simulink model "ROCAUC_2016b"  (R2016b)
settings: Solver=VariableStepAuto  StartTime=0.0  StopTime=10.0  RelTol=1e-3
settings Model: Creator=aoki-soya  LastModifiedBy=aoki-soya

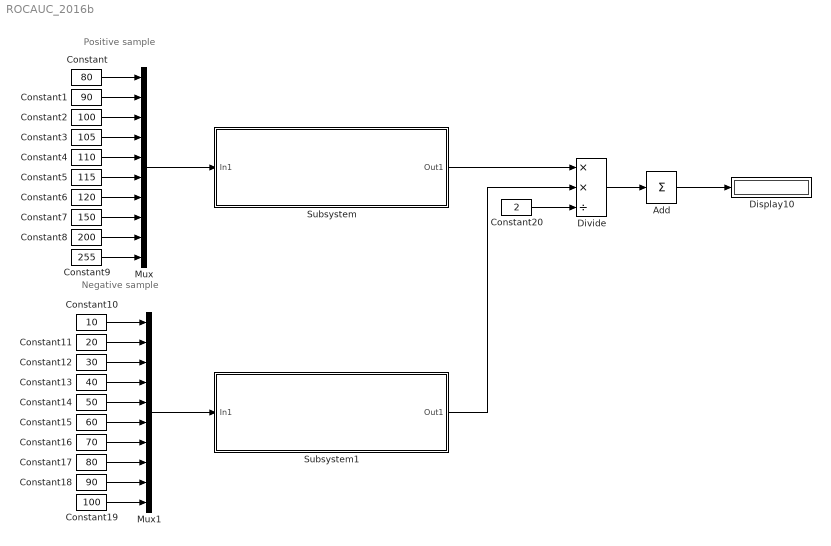
== system ROCAUC_2016b ==
  note: Positive sample
  note: Negative sample
  Add : Sum  Inputs=+
  Constant : Constant  Value=80
  Constant1 : Constant  Value=90
  Constant10 : Constant  Value=10
  Constant11 : Constant  Value=20
  Constant12 : Constant  Value=30
  Constant13 : Constant  Value=40
  Constant14 : Constant  Value=50
  Constant15 : Constant  Value=60
  Constant16 : Constant  Value=70
  Constant17 : Constant  Value=80
  Constant18 : Constant  Value=90
  Constant19 : Constant  Value=100
  Constant2 : Constant  Value=100
  Constant20 : Constant  Value=2
  Constant3 : Constant  Value=105
  Constant4 : Constant  Value=110
  Constant5 : Constant  Value=115
  Constant6 : Constant  Value=120
  Constant7 : Constant  Value=150
  Constant8 : Constant  Value=200
  Constant9 : Constant  Value=255
  Display10 : Display
  Divide : Product  Inputs=**/
  Mux : Mux  Inputs=10
  Mux1 : Mux  Inputs=10
  Subsystem : Subsystem
  Subsystem1 : Subsystem
  wires:
  Constant/1 -> Mux/1
  Constant2/1 -> Mux/3
  Constant1/1 -> Mux/2
  Constant3/1 -> Mux/4
  Constant4/1 -> Mux/5
  Constant5/1 -> Mux/6
  Constant6/1 -> Mux/7
  Constant7/1 -> Mux/8
  Constant8/1 -> Mux/9
  Constant9/1 -> Mux/10
  Constant10/1 -> Mux1/1
  Constant14/1 -> Mux1/5
  Constant13/1 -> Mux1/4
  Constant18/1 -> Mux1/9
  Constant15/1 -> Mux1/6
  Constant16/1 -> Mux1/7
  Constant17/1 -> Mux1/8
  Constant19/1 -> Mux1/10
  Constant11/1 -> Mux1/2
  Constant12/1 -> Mux1/3
  Constant20/1 -> Divide/3
  Mux/1 -> Subsystem/1(In1)
  Mux1/1 -> Subsystem1/1(In1)
  Subsystem/1(Out1) -> Divide/1
  Subsystem1/1(Out1) -> Divide/2
  Divide/1 -> Add/1
  Add/1 -> Display10/1

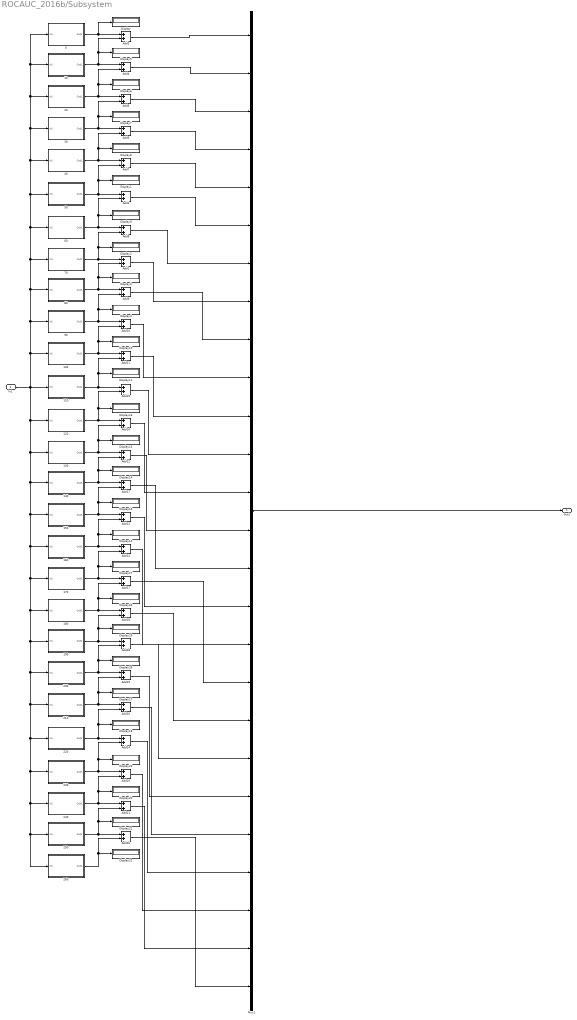
== system ROCAUC_2016b/Subsystem ==
  In1 : Inport
  0 : Subsystem
  10 : Subsystem
  100 : Subsystem
  110 : Subsystem
  120 : Subsystem
  130 : Subsystem
  140 : Subsystem
  150 : Subsystem
  160 : Subsystem
  170 : Subsystem
  180 : Subsystem
  190 : Subsystem
  20 : Subsystem
  200 : Subsystem
  210 : Subsystem
  220 : Subsystem
  230 : Subsystem
  240 : Subsystem
  250 : Subsystem
  260 : Subsystem
  30 : Subsystem
  40 : Subsystem
  50 : Subsystem
  60 : Subsystem
  70 : Subsystem
  80 : Subsystem
  90 : Subsystem
  Add{1..21,24..28} (26 alike) : Sum
  Display{,1..18,20..27} (27 alike) : Display
  Mux2 : Mux  Inputs=26
  Out1 : Outport
  wires:
  0/1(Out1) -> Add3/1, Display/1
  Mux2/1 -> Out1/1
  Add3/1 -> Mux2/1
  50/1(Out1) -> Add7/2, Display1/1, Add2/1
  10/1(Out1) -> Add4/1, Display5/1, Add3/2
  Add4/1 -> Mux2/2
  20/1(Out1) -> Add5/1, Add4/2, Display6/1
  Add5/1 -> Mux2/3
  30/1(Out1) -> Add6/1, Add5/2, Display7/1
  Add6/1 -> Mux2/4
  40/1(Out1) -> Add7/1, Add6/2, Display8/1
  Add7/1 -> Mux2/5
  Add2/1 -> Mux2/6
  60/1(Out1) -> Add8/1, Add2/2, Display9/1
  Add8/1 -> Mux2/7
  90/1(Out1) -> Add10/1, Add9/2, Display4/1
  70/1(Out1) -> Add1/1, Display2/1, Add8/2
  80/1(Out1) -> Add9/1, Display3/1, Add1/2
  100/1(Out1) -> Add11/1, Add10/2, Display10/1
  Add1/1 -> Mux2/8
  Add9/1 -> Mux2/9
  Add10/1 -> Mux2/10
  Add11/1 -> Mux2/11
  130/1(Out1) -> Add12/1, Display13/1, Add16/2
  140/1(Out1) -> Add17/1, Display14/1, Add12/2
  110/1(Out1) -> Add11/2, Display11/1, Add15/1
  160/1(Out1) -> Add14/1, Add13/2, Display12/1
  150/1(Out1) -> Add13/1, Add17/2, Display15/1
  120/1(Out1) -> Add16/1, Add15/2, Display16/1
  Add15/1 -> Mux2/12
  Add16/1 -> Mux2/13
  Add12/1 -> Mux2/14
  Add17/1 -> Mux2/15
  Add13/1 -> Mux2/16
  Add14/1 -> Mux2/17
  210/1(Out1) -> Add20/1, Add19/2, Display17/1
  180/1(Out1) -> Add18/1, Display24/1, Add27/2
  In1/1 -> 260/1(In1), 250/1(In1), 240/1(In1), 230/1(In1), 220/1(In1), 210/1(In1), 200/1(In1), 190/1(In1), 180/1(In1), 170/1(In1), 160/1(In1), 150/1(In1), 140/1(In1), 130/1(In1), 120/1(In1), 100/1(In1), 90/1(In1), 80/1(In1), 70/1(In1), 60/1(In1), 40/1(In1), 30/1(In1), 20/1(In1), 10/1(In1), 0/1(In1), 50/1(In1), 110/1(In1)
  190/1(Out1) -> Add28/1, Display25/1, Add18/2
  240/1(Out1) -> Add21/1, Display20/1, Add25/2
  200/1(Out1) -> Add19/1, Add28/2, Display26/1
  260/1(Out1) -> Add26/2, Display22/1
  220/1(Out1) -> Add20/2, Display18/1, Add24/1
  230/1(Out1) -> Add25/1, Add24/2, Display23/1
  250/1(Out1) -> Add26/1, Display21/1, Add21/2
  170/1(Out1) -> Add27/1, Add14/2, Display27/1
  Add27/1 -> Mux2/18
  Add18/1 -> Mux2/19
  Add28/1 -> Mux2/20
  Add19/1 -> Mux2/21
  Add26/1 -> Mux2/26
  Add21/1 -> Mux2/25
  Add25/1 -> Mux2/24
  Add24/1 -> Mux2/23
  Add20/1 -> Mux2/22

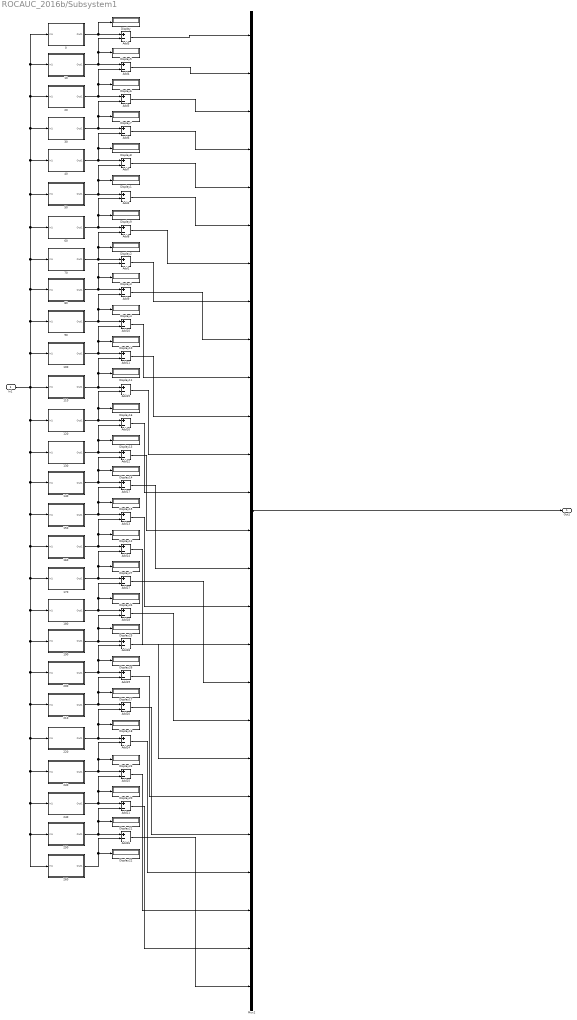
== system ROCAUC_2016b/Subsystem1 ==
  In1 : Inport
  0 : Subsystem
  10 : Subsystem
  100 : Subsystem
  110 : Subsystem
  120 : Subsystem
  130 : Subsystem
  140 : Subsystem
  150 : Subsystem
  160 : Subsystem
  170 : Subsystem
  180 : Subsystem
  190 : Subsystem
  20 : Subsystem
  200 : Subsystem
  210 : Subsystem
  220 : Subsystem
  230 : Subsystem
  240 : Subsystem
  250 : Subsystem
  260 : Subsystem
  30 : Subsystem
  40 : Subsystem
  50 : Subsystem
  60 : Subsystem
  70 : Subsystem
  80 : Subsystem
  90 : Subsystem
  Add{1..21,24..28} (26 alike) : Sum  Inputs=+-
  Display{,1..18,20..27} (27 alike) : Display
  Mux2 : Mux  Inputs=26
  Out1 : Outport
  wires:
  0/1(Out1) -> Add3/1, Display/1
  Mux2/1 -> Out1/1
  Add3/1 -> Mux2/1
  50/1(Out1) -> Add7/2, Display1/1, Add2/1
  10/1(Out1) -> Add4/1, Display5/1, Add3/2
  Add4/1 -> Mux2/2
  20/1(Out1) -> Add5/1, Add4/2, Display6/1
  Add5/1 -> Mux2/3
  30/1(Out1) -> Add6/1, Add5/2, Display7/1
  Add6/1 -> Mux2/4
  40/1(Out1) -> Add7/1, Add6/2, Display8/1
  Add7/1 -> Mux2/5
  Add2/1 -> Mux2/6
  60/1(Out1) -> Add8/1, Add2/2, Display9/1
  Add8/1 -> Mux2/7
  90/1(Out1) -> Add10/1, Add9/2, Display4/1
  70/1(Out1) -> Add1/1, Display2/1, Add8/2
  80/1(Out1) -> Add9/1, Display3/1, Add1/2
  100/1(Out1) -> Add11/1, Add10/2, Display10/1
  Add1/1 -> Mux2/8
  Add9/1 -> Mux2/9
  Add10/1 -> Mux2/10
  Add11/1 -> Mux2/11
  130/1(Out1) -> Add12/1, Display13/1, Add16/2
  140/1(Out1) -> Add17/1, Display14/1, Add12/2
  110/1(Out1) -> Add11/2, Display11/1, Add15/1
  160/1(Out1) -> Add14/1, Add13/2, Display12/1
  150/1(Out1) -> Add13/1, Add17/2, Display15/1
  120/1(Out1) -> Add16/1, Add15/2, Display16/1
  Add15/1 -> Mux2/12
  Add16/1 -> Mux2/13
  Add12/1 -> Mux2/14
  Add17/1 -> Mux2/15
  Add13/1 -> Mux2/16
  Add14/1 -> Mux2/17
  210/1(Out1) -> Add20/1, Add19/2, Display17/1
  180/1(Out1) -> Add18/1, Display24/1, Add27/2
  In1/1 -> 260/1(In1), 250/1(In1), 240/1(In1), 230/1(In1), 220/1(In1), 210/1(In1), 200/1(In1), 190/1(In1), 180/1(In1), 170/1(In1), 160/1(In1), 150/1(In1), 140/1(In1), 130/1(In1), 120/1(In1), 100/1(In1), 90/1(In1), 80/1(In1), 70/1(In1), 60/1(In1), 40/1(In1), 30/1(In1), 20/1(In1), 10/1(In1), 0/1(In1), 50/1(In1), 110/1(In1)
  190/1(Out1) -> Add28/1, Display25/1, Add18/2
  240/1(Out1) -> Add21/1, Display20/1, Add25/2
  200/1(Out1) -> Add19/1, Add28/2, Display26/1
  260/1(Out1) -> Add26/2, Display22/1
  220/1(Out1) -> Add20/2, Display18/1, Add24/1
  230/1(Out1) -> Add25/1, Add24/2, Display23/1
  250/1(Out1) -> Add26/1, Display21/1, Add21/2
  170/1(Out1) -> Add27/1, Add14/2, Display27/1
  Add27/1 -> Mux2/18
  Add18/1 -> Mux2/19
  Add28/1 -> Mux2/20
  Add19/1 -> Mux2/21
  Add26/1 -> Mux2/26
  Add21/1 -> Mux2/25
  Add25/1 -> Mux2/24
  Add24/1 -> Mux2/23
  Add20/1 -> Mux2/22

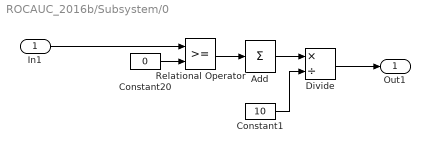
== system ROCAUC_2016b/Subsystem/0 ==
  In1 : Inport
  Add : Sum  Inputs=+
  Constant1 : Constant  Value=10
  Constant20 : Constant  Value=0
  Divide : Product  Inputs=*/
  Relational Operator : RelationalOperator  OutDataTypeStr=boolean  RndMeth=Simplest
  Out1 : Outport
  wires:
  Constant20/1 -> Relational Operator/2
  Relational Operator/1 -> Add/1
  In1/1 -> Relational Operator/1
  Add/1 -> Divide/1
  Divide/1 -> Out1/1
  Constant1/1 -> Divide/2

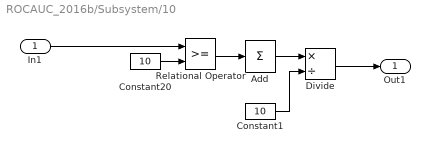
== system ROCAUC_2016b/Subsystem/10 ==
  In1 : Inport
  Add : Sum  Inputs=+
  Constant1 : Constant  Value=10
  Constant20 : Constant  Value=10
  Divide : Product  Inputs=*/
  Relational Operator : RelationalOperator  OutDataTypeStr=boolean  RndMeth=Simplest
  Out1 : Outport
  wires:
  Constant20/1 -> Relational Operator/2
  Relational Operator/1 -> Add/1
  In1/1 -> Relational Operator/1
  Add/1 -> Divide/1
  Divide/1 -> Out1/1
  Constant1/1 -> Divide/2

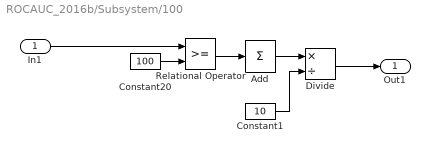
== system ROCAUC_2016b/Subsystem/100 ==
  In1 : Inport
  Add : Sum  Inputs=+
  Constant1 : Constant  Value=10
  Constant20 : Constant  Value=100
  Divide : Product  Inputs=*/
  Relational Operator : RelationalOperator  OutDataTypeStr=boolean  RndMeth=Simplest
  Out1 : Outport
  wires:
  Constant20/1 -> Relational Operator/2
  Relational Operator/1 -> Add/1
  In1/1 -> Relational Operator/1
  Add/1 -> Divide/1
  Divide/1 -> Out1/1
  Constant1/1 -> Divide/2

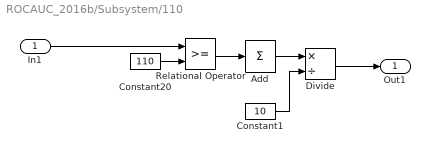
== system ROCAUC_2016b/Subsystem/110 ==
  In1 : Inport
  Add : Sum  Inputs=+
  Constant1 : Constant  Value=10
  Constant20 : Constant  Value=110
  Divide : Product  Inputs=*/
  Relational Operator : RelationalOperator  OutDataTypeStr=boolean  RndMeth=Simplest
  Out1 : Outport
  wires:
  In1/1 -> Relational Operator/1
  Relational Operator/1 -> Add/1
  Constant1/1 -> Divide/2
  Add/1 -> Divide/1
  Constant20/1 -> Relational Operator/2
  Divide/1 -> Out1/1

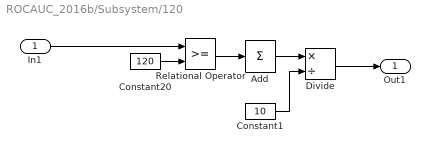
== system ROCAUC_2016b/Subsystem/120 ==
  In1 : Inport
  Add : Sum  Inputs=+
  Constant1 : Constant  Value=10
  Constant20 : Constant  Value=120
  Divide : Product  Inputs=*/
  Relational Operator : RelationalOperator  OutDataTypeStr=boolean  RndMeth=Simplest
  Out1 : Outport
  wires:
  Constant20/1 -> Relational Operator/2
  Relational Operator/1 -> Add/1
  In1/1 -> Relational Operator/1
  Add/1 -> Divide/1
  Divide/1 -> Out1/1
  Constant1/1 -> Divide/2

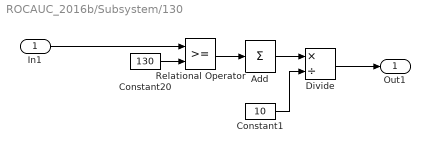
== system ROCAUC_2016b/Subsystem/130 ==
  In1 : Inport
  Add : Sum  Inputs=+
  Constant1 : Constant  Value=10
  Constant20 : Constant  Value=130
  Divide : Product  Inputs=*/
  Relational Operator : RelationalOperator  OutDataTypeStr=boolean  RndMeth=Simplest
  Out1 : Outport
  wires:
  Constant20/1 -> Relational Operator/2
  Relational Operator/1 -> Add/1
  In1/1 -> Relational Operator/1
  Add/1 -> Divide/1
  Divide/1 -> Out1/1
  Constant1/1 -> Divide/2

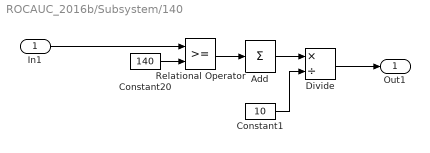
== system ROCAUC_2016b/Subsystem/140 ==
  In1 : Inport
  Add : Sum  Inputs=+
  Constant1 : Constant  Value=10
  Constant20 : Constant  Value=140
  Divide : Product  Inputs=*/
  Relational Operator : RelationalOperator  OutDataTypeStr=boolean  RndMeth=Simplest
  Out1 : Outport
  wires:
  Constant20/1 -> Relational Operator/2
  Relational Operator/1 -> Add/1
  In1/1 -> Relational Operator/1
  Add/1 -> Divide/1
  Divide/1 -> Out1/1
  Constant1/1 -> Divide/2

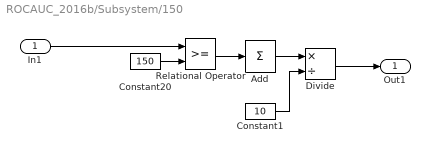
== system ROCAUC_2016b/Subsystem/150 ==
  In1 : Inport
  Add : Sum  Inputs=+
  Constant1 : Constant  Value=10
  Constant20 : Constant  Value=150
  Divide : Product  Inputs=*/
  Relational Operator : RelationalOperator  OutDataTypeStr=boolean  RndMeth=Simplest
  Out1 : Outport
  wires:
  Constant20/1 -> Relational Operator/2
  Relational Operator/1 -> Add/1
  In1/1 -> Relational Operator/1
  Add/1 -> Divide/1
  Divide/1 -> Out1/1
  Constant1/1 -> Divide/2

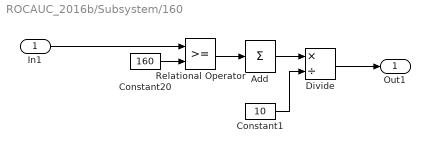
== system ROCAUC_2016b/Subsystem/160 ==
  In1 : Inport
  Add : Sum  Inputs=+
  Constant1 : Constant  Value=10
  Constant20 : Constant  Value=160
  Divide : Product  Inputs=*/
  Relational Operator : RelationalOperator  OutDataTypeStr=boolean  RndMeth=Simplest
  Out1 : Outport
  wires:
  Constant20/1 -> Relational Operator/2
  Relational Operator/1 -> Add/1
  In1/1 -> Relational Operator/1
  Add/1 -> Divide/1
  Divide/1 -> Out1/1
  Constant1/1 -> Divide/2

== system ROCAUC_2016b/Subsystem/170 ==
  In1 : Inport
  Add : Sum  Inputs=+
  Constant1 : Constant  Value=10
  Constant20 : Constant  Value=170
  Divide : Product  Inputs=*/
  Relational Operator : RelationalOperator  OutDataTypeStr=boolean  RndMeth=Simplest
  Out1 : Outport
  wires:
  Constant20/1 -> Relational Operator/2
  Relational Operator/1 -> Add/1
  In1/1 -> Relational Operator/1
  Add/1 -> Divide/1
  Divide/1 -> Out1/1
  Constant1/1 -> Divide/2

== system ROCAUC_2016b/Subsystem/180 ==
  In1 : Inport
  Add : Sum  Inputs=+
  Constant1 : Constant  Value=10
  Constant20 : Constant  Value=180
  Divide : Product  Inputs=*/
  Relational Operator : RelationalOperator  OutDataTypeStr=boolean  RndMeth=Simplest
  Out1 : Outport
  wires:
  Constant20/1 -> Relational Operator/2
  Relational Operator/1 -> Add/1
  In1/1 -> Relational Operator/1
  Add/1 -> Divide/1
  Divide/1 -> Out1/1
  Constant1/1 -> Divide/2

== system ROCAUC_2016b/Subsystem/190 ==
  In1 : Inport
  Add : Sum  Inputs=+
  Constant1 : Constant  Value=10
  Constant20 : Constant  Value=190
  Divide : Product  Inputs=*/
  Relational Operator : RelationalOperator  OutDataTypeStr=boolean  RndMeth=Simplest
  Out1 : Outport
  wires:
  Constant20/1 -> Relational Operator/2
  Relational Operator/1 -> Add/1
  In1/1 -> Relational Operator/1
  Add/1 -> Divide/1
  Divide/1 -> Out1/1
  Constant1/1 -> Divide/2

== system ROCAUC_2016b/Subsystem/20 ==
  In1 : Inport
  Add : Sum  Inputs=+
  Constant1 : Constant  Value=10
  Constant20 : Constant  Value=20
  Divide : Product  Inputs=*/
  Relational Operator : RelationalOperator  OutDataTypeStr=boolean  RndMeth=Simplest
  Out1 : Outport
  wires:
  Constant20/1 -> Relational Operator/2
  Relational Operator/1 -> Add/1
  In1/1 -> Relational Operator/1
  Add/1 -> Divide/1
  Divide/1 -> Out1/1
  Constant1/1 -> Divide/2

== system ROCAUC_2016b/Subsystem/200 ==
  In1 : Inport
  Add : Sum  Inputs=+
  Constant1 : Constant  Value=10
  Constant20 : Constant  Value=200
  Divide : Product  Inputs=*/
  Relational Operator : RelationalOperator  OutDataTypeStr=boolean  RndMeth=Simplest
  Out1 : Outport
  wires:
  Constant20/1 -> Relational Operator/2
  Relational Operator/1 -> Add/1
  In1/1 -> Relational Operator/1
  Add/1 -> Divide/1
  Divide/1 -> Out1/1
  Constant1/1 -> Divide/2

== system ROCAUC_2016b/Subsystem/210 ==
  In1 : Inport
  Add : Sum  Inputs=+
  Constant1 : Constant  Value=10
  Constant20 : Constant  Value=210
  Divide : Product  Inputs=*/
  Relational Operator : RelationalOperator  OutDataTypeStr=boolean  RndMeth=Simplest
  Out1 : Outport
  wires:
  Constant20/1 -> Relational Operator/2
  Relational Operator/1 -> Add/1
  In1/1 -> Relational Operator/1
  Add/1 -> Divide/1
  Divide/1 -> Out1/1
  Constant1/1 -> Divide/2

== system ROCAUC_2016b/Subsystem/220 ==
  In1 : Inport
  Add : Sum  Inputs=+
  Constant1 : Constant  Value=10
  Constant20 : Constant  Value=220
  Divide : Product  Inputs=*/
  Relational Operator : RelationalOperator  OutDataTypeStr=boolean  RndMeth=Simplest
  Out1 : Outport
  wires:
  In1/1 -> Relational Operator/1
  Relational Operator/1 -> Add/1
  Constant1/1 -> Divide/2
  Add/1 -> Divide/1
  Constant20/1 -> Relational Operator/2
  Divide/1 -> Out1/1

== system ROCAUC_2016b/Subsystem/230 ==
  In1 : Inport
  Add : Sum  Inputs=+
  Constant1 : Constant  Value=10
  Constant20 : Constant  Value=230
  Divide : Product  Inputs=*/
  Relational Operator : RelationalOperator  OutDataTypeStr=boolean  RndMeth=Simplest
  Out1 : Outport
  wires:
  Constant20/1 -> Relational Operator/2
  Relational Operator/1 -> Add/1
  In1/1 -> Relational Operator/1
  Add/1 -> Divide/1
  Divide/1 -> Out1/1
  Constant1/1 -> Divide/2

== system ROCAUC_2016b/Subsystem/240 ==
  In1 : Inport
  Add : Sum  Inputs=+
  Constant1 : Constant  Value=10
  Constant20 : Constant  Value=240
  Divide : Product  Inputs=*/
  Relational Operator : RelationalOperator  OutDataTypeStr=boolean  RndMeth=Simplest
  Out1 : Outport
  wires:
  Constant20/1 -> Relational Operator/2
  Relational Operator/1 -> Add/1
  In1/1 -> Relational Operator/1
  Add/1 -> Divide/1
  Divide/1 -> Out1/1
  Constant1/1 -> Divide/2

== system ROCAUC_2016b/Subsystem/250 ==
  In1 : Inport
  Add : Sum  Inputs=+
  Constant1 : Constant  Value=10
  Constant20 : Constant  Value=250
  Divide : Product  Inputs=*/
  Relational Operator : RelationalOperator  OutDataTypeStr=boolean  RndMeth=Simplest
  Out1 : Outport
  wires:
  Constant20/1 -> Relational Operator/2
  Relational Operator/1 -> Add/1
  In1/1 -> Relational Operator/1
  Add/1 -> Divide/1
  Divide/1 -> Out1/1
  Constant1/1 -> Divide/2

== system ROCAUC_2016b/Subsystem/260 ==
  In1 : Inport
  Add : Sum  Inputs=+
  Constant1 : Constant  Value=10
  Constant20 : Constant  Value=260
  Divide : Product  Inputs=*/
  Relational Operator : RelationalOperator  OutDataTypeStr=boolean  RndMeth=Simplest
  Out1 : Outport
  wires:
  Constant20/1 -> Relational Operator/2
  Relational Operator/1 -> Add/1
  In1/1 -> Relational Operator/1
  Add/1 -> Divide/1
  Divide/1 -> Out1/1
  Constant1/1 -> Divide/2

== system ROCAUC_2016b/Subsystem/30 ==
  In1 : Inport
  Add : Sum  Inputs=+
  Constant1 : Constant  Value=10
  Constant20 : Constant  Value=30
  Divide : Product  Inputs=*/
  Relational Operator : RelationalOperator  OutDataTypeStr=boolean  RndMeth=Simplest
  Out1 : Outport
  wires:
  Constant20/1 -> Relational Operator/2
  Relational Operator/1 -> Add/1
  In1/1 -> Relational Operator/1
  Add/1 -> Divide/1
  Divide/1 -> Out1/1
  Constant1/1 -> Divide/2

== system ROCAUC_2016b/Subsystem/40 ==
  In1 : Inport
  Add : Sum  Inputs=+
  Constant1 : Constant  Value=10
  Constant20 : Constant  Value=40
  Divide : Product  Inputs=*/
  Relational Operator : RelationalOperator  OutDataTypeStr=boolean  RndMeth=Simplest
  Out1 : Outport
  wires:
  Constant20/1 -> Relational Operator/2
  Relational Operator/1 -> Add/1
  In1/1 -> Relational Operator/1
  Add/1 -> Divide/1
  Divide/1 -> Out1/1
  Constant1/1 -> Divide/2

== system ROCAUC_2016b/Subsystem/50 ==
  In1 : Inport
  Add : Sum  Inputs=+
  Constant1 : Constant  Value=10
  Constant20 : Constant  Value=50
  Divide : Product  Inputs=*/
  Relational Operator : RelationalOperator  OutDataTypeStr=boolean  RndMeth=Simplest
  Out1 : Outport
  wires:
  In1/1 -> Relational Operator/1
  Relational Operator/1 -> Add/1
  Constant1/1 -> Divide/2
  Add/1 -> Divide/1
  Constant20/1 -> Relational Operator/2
  Divide/1 -> Out1/1

== system ROCAUC_2016b/Subsystem/60 ==
  In1 : Inport
  Add : Sum  Inputs=+
  Constant1 : Constant  Value=10
  Constant20 : Constant  Value=60
  Divide : Product  Inputs=*/
  Relational Operator : RelationalOperator  OutDataTypeStr=boolean  RndMeth=Simplest
  Out1 : Outport
  wires:
  Constant20/1 -> Relational Operator/2
  Relational Operator/1 -> Add/1
  In1/1 -> Relational Operator/1
  Add/1 -> Divide/1
  Divide/1 -> Out1/1
  Constant1/1 -> Divide/2

== system ROCAUC_2016b/Subsystem/70 ==
  In1 : Inport
  Add : Sum  Inputs=+
  Constant1 : Constant  Value=10
  Constant20 : Constant  Value=70
  Divide : Product  Inputs=*/
  Relational Operator : RelationalOperator  OutDataTypeStr=boolean  RndMeth=Simplest
  Out1 : Outport
  wires:
  Constant20/1 -> Relational Operator/2
  Relational Operator/1 -> Add/1
  In1/1 -> Relational Operator/1
  Add/1 -> Divide/1
  Divide/1 -> Out1/1
  Constant1/1 -> Divide/2

== system ROCAUC_2016b/Subsystem/80 ==
  In1 : Inport
  Add : Sum  Inputs=+
  Constant1 : Constant  Value=10
  Constant20 : Constant  Value=80
  Divide : Product  Inputs=*/
  Relational Operator : RelationalOperator  OutDataTypeStr=boolean  RndMeth=Simplest
  Out1 : Outport
  wires:
  Constant20/1 -> Relational Operator/2
  Relational Operator/1 -> Add/1
  In1/1 -> Relational Operator/1
  Add/1 -> Divide/1
  Divide/1 -> Out1/1
  Constant1/1 -> Divide/2

== system ROCAUC_2016b/Subsystem/90 ==
  In1 : Inport
  Add : Sum  Inputs=+
  Constant1 : Constant  Value=10
  Constant20 : Constant  Value=90
  Divide : Product  Inputs=*/
  Relational Operator : RelationalOperator  OutDataTypeStr=boolean  RndMeth=Simplest
  Out1 : Outport
  wires:
  Constant20/1 -> Relational Operator/2
  Relational Operator/1 -> Add/1
  In1/1 -> Relational Operator/1
  Add/1 -> Divide/1
  Divide/1 -> Out1/1
  Constant1/1 -> Divide/2

== system ROCAUC_2016b/Subsystem1/0 ==
  In1 : Inport
  Add : Sum  Inputs=+
  Constant1 : Constant  Value=10
  Constant20 : Constant  Value=0
  Divide : Product  Inputs=*/
  Relational Operator : RelationalOperator  OutDataTypeStr=boolean  RndMeth=Simplest
  Out1 : Outport
  wires:
  Constant20/1 -> Relational Operator/2
  Relational Operator/1 -> Add/1
  In1/1 -> Relational Operator/1
  Add/1 -> Divide/1
  Divide/1 -> Out1/1
  Constant1/1 -> Divide/2

== system ROCAUC_2016b/Subsystem1/10 ==
  In1 : Inport
  Add : Sum  Inputs=+
  Constant1 : Constant  Value=10
  Constant20 : Constant  Value=10
  Divide : Product  Inputs=*/
  Relational Operator : RelationalOperator  OutDataTypeStr=boolean  RndMeth=Simplest
  Out1 : Outport
  wires:
  Constant20/1 -> Relational Operator/2
  Relational Operator/1 -> Add/1
  In1/1 -> Relational Operator/1
  Add/1 -> Divide/1
  Divide/1 -> Out1/1
  Constant1/1 -> Divide/2

== system ROCAUC_2016b/Subsystem1/100 ==
  In1 : Inport
  Add : Sum  Inputs=+
  Constant1 : Constant  Value=10
  Constant20 : Constant  Value=100
  Divide : Product  Inputs=*/
  Relational Operator : RelationalOperator  OutDataTypeStr=boolean  RndMeth=Simplest
  Out1 : Outport
  wires:
  Constant20/1 -> Relational Operator/2
  Relational Operator/1 -> Add/1
  In1/1 -> Relational Operator/1
  Add/1 -> Divide/1
  Divide/1 -> Out1/1
  Constant1/1 -> Divide/2

== system ROCAUC_2016b/Subsystem1/110 ==
  In1 : Inport
  Add : Sum  Inputs=+
  Constant1 : Constant  Value=10
  Constant20 : Constant  Value=110
  Divide : Product  Inputs=*/
  Relational Operator : RelationalOperator  OutDataTypeStr=boolean  RndMeth=Simplest
  Out1 : Outport
  wires:
  In1/1 -> Relational Operator/1
  Relational Operator/1 -> Add/1
  Constant1/1 -> Divide/2
  Add/1 -> Divide/1
  Constant20/1 -> Relational Operator/2
  Divide/1 -> Out1/1

== system ROCAUC_2016b/Subsystem1/120 ==
  In1 : Inport
  Add : Sum  Inputs=+
  Constant1 : Constant  Value=10
  Constant20 : Constant  Value=120
  Divide : Product  Inputs=*/
  Relational Operator : RelationalOperator  OutDataTypeStr=boolean  RndMeth=Simplest
  Out1 : Outport
  wires:
  Constant20/1 -> Relational Operator/2
  Relational Operator/1 -> Add/1
  In1/1 -> Relational Operator/1
  Add/1 -> Divide/1
  Divide/1 -> Out1/1
  Constant1/1 -> Divide/2

== system ROCAUC_2016b/Subsystem1/130 ==
  In1 : Inport
  Add : Sum  Inputs=+
  Constant1 : Constant  Value=10
  Constant20 : Constant  Value=130
  Divide : Product  Inputs=*/
  Relational Operator : RelationalOperator  OutDataTypeStr=boolean  RndMeth=Simplest
  Out1 : Outport
  wires:
  Constant20/1 -> Relational Operator/2
  Relational Operator/1 -> Add/1
  In1/1 -> Relational Operator/1
  Add/1 -> Divide/1
  Divide/1 -> Out1/1
  Constant1/1 -> Divide/2

== system ROCAUC_2016b/Subsystem1/140 ==
  In1 : Inport
  Add : Sum  Inputs=+
  Constant1 : Constant  Value=10
  Constant20 : Constant  Value=140
  Divide : Product  Inputs=*/
  Relational Operator : RelationalOperator  OutDataTypeStr=boolean  RndMeth=Simplest
  Out1 : Outport
  wires:
  Constant20/1 -> Relational Operator/2
  Relational Operator/1 -> Add/1
  In1/1 -> Relational Operator/1
  Add/1 -> Divide/1
  Divide/1 -> Out1/1
  Constant1/1 -> Divide/2

== system ROCAUC_2016b/Subsystem1/150 ==
  In1 : Inport
  Add : Sum  Inputs=+
  Constant1 : Constant  Value=10
  Constant20 : Constant  Value=150
  Divide : Product  Inputs=*/
  Relational Operator : RelationalOperator  OutDataTypeStr=boolean  RndMeth=Simplest
  Out1 : Outport
  wires:
  Constant20/1 -> Relational Operator/2
  Relational Operator/1 -> Add/1
  In1/1 -> Relational Operator/1
  Add/1 -> Divide/1
  Divide/1 -> Out1/1
  Constant1/1 -> Divide/2

== system ROCAUC_2016b/Subsystem1/160 ==
  In1 : Inport
  Add : Sum  Inputs=+
  Constant1 : Constant  Value=10
  Constant20 : Constant  Value=160
  Divide : Product  Inputs=*/
  Relational Operator : RelationalOperator  OutDataTypeStr=boolean  RndMeth=Simplest
  Out1 : Outport
  wires:
  Constant20/1 -> Relational Operator/2
  Relational Operator/1 -> Add/1
  In1/1 -> Relational Operator/1
  Add/1 -> Divide/1
  Divide/1 -> Out1/1
  Constant1/1 -> Divide/2

== system ROCAUC_2016b/Subsystem1/170 ==
  In1 : Inport
  Add : Sum  Inputs=+
  Constant1 : Constant  Value=10
  Constant20 : Constant  Value=170
  Divide : Product  Inputs=*/
  Relational Operator : RelationalOperator  OutDataTypeStr=boolean  RndMeth=Simplest
  Out1 : Outport
  wires:
  Constant20/1 -> Relational Operator/2
  Relational Operator/1 -> Add/1
  In1/1 -> Relational Operator/1
  Add/1 -> Divide/1
  Divide/1 -> Out1/1
  Constant1/1 -> Divide/2

== system ROCAUC_2016b/Subsystem1/180 ==
  In1 : Inport
  Add : Sum  Inputs=+
  Constant1 : Constant  Value=10
  Constant20 : Constant  Value=180
  Divide : Product  Inputs=*/
  Relational Operator : RelationalOperator  OutDataTypeStr=boolean  RndMeth=Simplest
  Out1 : Outport
  wires:
  Constant20/1 -> Relational Operator/2
  Relational Operator/1 -> Add/1
  In1/1 -> Relational Operator/1
  Add/1 -> Divide/1
  Divide/1 -> Out1/1
  Constant1/1 -> Divide/2

== system ROCAUC_2016b/Subsystem1/190 ==
  In1 : Inport
  Add : Sum  Inputs=+
  Constant1 : Constant  Value=10
  Constant20 : Constant  Value=190
  Divide : Product  Inputs=*/
  Relational Operator : RelationalOperator  OutDataTypeStr=boolean  RndMeth=Simplest
  Out1 : Outport
  wires:
  Constant20/1 -> Relational Operator/2
  Relational Operator/1 -> Add/1
  In1/1 -> Relational Operator/1
  Add/1 -> Divide/1
  Divide/1 -> Out1/1
  Constant1/1 -> Divide/2

== system ROCAUC_2016b/Subsystem1/20 ==
  In1 : Inport
  Add : Sum  Inputs=+
  Constant1 : Constant  Value=10
  Constant20 : Constant  Value=20
  Divide : Product  Inputs=*/
  Relational Operator : RelationalOperator  OutDataTypeStr=boolean  RndMeth=Simplest
  Out1 : Outport
  wires:
  Constant20/1 -> Relational Operator/2
  Relational Operator/1 -> Add/1
  In1/1 -> Relational Operator/1
  Add/1 -> Divide/1
  Divide/1 -> Out1/1
  Constant1/1 -> Divide/2

== system ROCAUC_2016b/Subsystem1/200 ==
  In1 : Inport
  Add : Sum  Inputs=+
  Constant1 : Constant  Value=10
  Constant20 : Constant  Value=200
  Divide : Product  Inputs=*/
  Relational Operator : RelationalOperator  OutDataTypeStr=boolean  RndMeth=Simplest
  Out1 : Outport
  wires:
  Constant20/1 -> Relational Operator/2
  Relational Operator/1 -> Add/1
  In1/1 -> Relational Operator/1
  Add/1 -> Divide/1
  Divide/1 -> Out1/1
  Constant1/1 -> Divide/2

== system ROCAUC_2016b/Subsystem1/210 ==
  In1 : Inport
  Add : Sum  Inputs=+
  Constant1 : Constant  Value=10
  Constant20 : Constant  Value=210
  Divide : Product  Inputs=*/
  Relational Operator : RelationalOperator  OutDataTypeStr=boolean  RndMeth=Simplest
  Out1 : Outport
  wires:
  Constant20/1 -> Relational Operator/2
  Relational Operator/1 -> Add/1
  In1/1 -> Relational Operator/1
  Add/1 -> Divide/1
  Divide/1 -> Out1/1
  Constant1/1 -> Divide/2

== system ROCAUC_2016b/Subsystem1/220 ==
  In1 : Inport
  Add : Sum  Inputs=+
  Constant1 : Constant  Value=10
  Constant20 : Constant  Value=220
  Divide : Product  Inputs=*/
  Relational Operator : RelationalOperator  OutDataTypeStr=boolean  RndMeth=Simplest
  Out1 : Outport
  wires:
  In1/1 -> Relational Operator/1
  Relational Operator/1 -> Add/1
  Constant1/1 -> Divide/2
  Add/1 -> Divide/1
  Constant20/1 -> Relational Operator/2
  Divide/1 -> Out1/1

== system ROCAUC_2016b/Subsystem1/230 ==
  In1 : Inport
  Add : Sum  Inputs=+
  Constant1 : Constant  Value=10
  Constant20 : Constant  Value=230
  Divide : Product  Inputs=*/
  Relational Operator : RelationalOperator  OutDataTypeStr=boolean  RndMeth=Simplest
  Out1 : Outport
  wires:
  Constant20/1 -> Relational Operator/2
  Relational Operator/1 -> Add/1
  In1/1 -> Relational Operator/1
  Add/1 -> Divide/1
  Divide/1 -> Out1/1
  Constant1/1 -> Divide/2

== system ROCAUC_2016b/Subsystem1/240 ==
  In1 : Inport
  Add : Sum  Inputs=+
  Constant1 : Constant  Value=10
  Constant20 : Constant  Value=240
  Divide : Product  Inputs=*/
  Relational Operator : RelationalOperator  OutDataTypeStr=boolean  RndMeth=Simplest
  Out1 : Outport
  wires:
  Constant20/1 -> Relational Operator/2
  Relational Operator/1 -> Add/1
  In1/1 -> Relational Operator/1
  Add/1 -> Divide/1
  Divide/1 -> Out1/1
  Constant1/1 -> Divide/2

== system ROCAUC_2016b/Subsystem1/250 ==
  In1 : Inport
  Add : Sum  Inputs=+
  Constant1 : Constant  Value=10
  Constant20 : Constant  Value=250
  Divide : Product  Inputs=*/
  Relational Operator : RelationalOperator  OutDataTypeStr=boolean  RndMeth=Simplest
  Out1 : Outport
  wires:
  Constant20/1 -> Relational Operator/2
  Relational Operator/1 -> Add/1
  In1/1 -> Relational Operator/1
  Add/1 -> Divide/1
  Divide/1 -> Out1/1
  Constant1/1 -> Divide/2

== system ROCAUC_2016b/Subsystem1/260 ==
  In1 : Inport
  Add : Sum  Inputs=+
  Constant1 : Constant  Value=10
  Constant20 : Constant  Value=260
  Divide : Product  Inputs=*/
  Relational Operator : RelationalOperator  OutDataTypeStr=boolean  RndMeth=Simplest
  Out1 : Outport
  wires:
  Constant20/1 -> Relational Operator/2
  Relational Operator/1 -> Add/1
  In1/1 -> Relational Operator/1
  Add/1 -> Divide/1
  Divide/1 -> Out1/1
  Constant1/1 -> Divide/2

== system ROCAUC_2016b/Subsystem1/30 ==
  In1 : Inport
  Add : Sum  Inputs=+
  Constant1 : Constant  Value=10
  Constant20 : Constant  Value=30
  Divide : Product  Inputs=*/
  Relational Operator : RelationalOperator  OutDataTypeStr=boolean  RndMeth=Simplest
  Out1 : Outport
  wires:
  Constant20/1 -> Relational Operator/2
  Relational Operator/1 -> Add/1
  In1/1 -> Relational Operator/1
  Add/1 -> Divide/1
  Divide/1 -> Out1/1
  Constant1/1 -> Divide/2

== system ROCAUC_2016b/Subsystem1/40 ==
  In1 : Inport
  Add : Sum  Inputs=+
  Constant1 : Constant  Value=10
  Constant20 : Constant  Value=40
  Divide : Product  Inputs=*/
  Relational Operator : RelationalOperator  OutDataTypeStr=boolean  RndMeth=Simplest
  Out1 : Outport
  wires:
  Constant20/1 -> Relational Operator/2
  Relational Operator/1 -> Add/1
  In1/1 -> Relational Operator/1
  Add/1 -> Divide/1
  Divide/1 -> Out1/1
  Constant1/1 -> Divide/2

== system ROCAUC_2016b/Subsystem1/50 ==
  In1 : Inport
  Add : Sum  Inputs=+
  Constant1 : Constant  Value=10
  Constant20 : Constant  Value=50
  Divide : Product  Inputs=*/
  Relational Operator : RelationalOperator  OutDataTypeStr=boolean  RndMeth=Simplest
  Out1 : Outport
  wires:
  In1/1 -> Relational Operator/1
  Relational Operator/1 -> Add/1
  Constant1/1 -> Divide/2
  Add/1 -> Divide/1
  Constant20/1 -> Relational Operator/2
  Divide/1 -> Out1/1

== system ROCAUC_2016b/Subsystem1/60 ==
  In1 : Inport
  Add : Sum  Inputs=+
  Constant1 : Constant  Value=10
  Constant20 : Constant  Value=60
  Divide : Product  Inputs=*/
  Relational Operator : RelationalOperator  OutDataTypeStr=boolean  RndMeth=Simplest
  Out1 : Outport
  wires:
  Constant20/1 -> Relational Operator/2
  Relational Operator/1 -> Add/1
  In1/1 -> Relational Operator/1
  Add/1 -> Divide/1
  Divide/1 -> Out1/1
  Constant1/1 -> Divide/2

== system ROCAUC_2016b/Subsystem1/70 ==
  In1 : Inport
  Add : Sum  Inputs=+
  Constant1 : Constant  Value=10
  Constant20 : Constant  Value=70
  Divide : Product  Inputs=*/
  Relational Operator : RelationalOperator  OutDataTypeStr=boolean  RndMeth=Simplest
  Out1 : Outport
  wires:
  Constant20/1 -> Relational Operator/2
  Relational Operator/1 -> Add/1
  In1/1 -> Relational Operator/1
  Add/1 -> Divide/1
  Divide/1 -> Out1/1
  Constant1/1 -> Divide/2

== system ROCAUC_2016b/Subsystem1/80 ==
  In1 : Inport
  Add : Sum  Inputs=+
  Constant1 : Constant  Value=10
  Constant20 : Constant  Value=80
  Divide : Product  Inputs=*/
  Relational Operator : RelationalOperator  OutDataTypeStr=boolean  RndMeth=Simplest
  Out1 : Outport
  wires:
  Constant20/1 -> Relational Operator/2
  Relational Operator/1 -> Add/1
  In1/1 -> Relational Operator/1
  Add/1 -> Divide/1
  Divide/1 -> Out1/1
  Constant1/1 -> Divide/2

== system ROCAUC_2016b/Subsystem1/90 ==
  In1 : Inport
  Add : Sum  Inputs=+
  Constant1 : Constant  Value=10
  Constant20 : Constant  Value=90
  Divide : Product  Inputs=*/
  Relational Operator : RelationalOperator  OutDataTypeStr=boolean  RndMeth=Simplest
  Out1 : Outport
  wires:
  Constant20/1 -> Relational Operator/2
  Relational Operator/1 -> Add/1
  In1/1 -> Relational Operator/1
  Add/1 -> Divide/1
  Divide/1 -> Out1/1
  Constant1/1 -> Divide/2
